simulink model "Problem16_BDsketch"  (R2020b)
settings: Solver=VariableStepAuto  StartTime=0.0  StopTime=10.0  RelTol=1e-3
values from neighbouring files (symbols this model uses):
  K_D = 2*zeta/omega_n * K_p - feff / kT    [problem12.m]    (also in problem13.m; problem15.m = (2*omega_n*zeta*tau_i + 1 - feff) ./ kT; problem16.m = (2*omega_n*zeta*tau_i + 1 - feff) ./ kT; problem17.m = (2*omega_n*zeta*tau_i + 1 - feff) ./ kT)
  K_I = omega_n^2 / kT    (= 1323.52941176)    [problem15.m]    (also in problem16.m = omega_n^2 / kT * ones(4,1); problem17.m = omega_n^2 / kT * ones(4,1); problem18.m; problem20.m = omega_n^2 / kT .* ones(4,1))
  kT = 0.17    [problem12.m]    (also in problem13.m; problem15.m; problem16.m; problem17.m)
  n = 53    [Problem7_9.m]    (also in Problem8_script.m = length(t); problem12.m; problem13.m; problem15.m)
undefined symbols (not defined in the file or in its folder): f_eff, J_eff, K_P
settings Model: Creator=Theis  LastModifiedBy=Theis

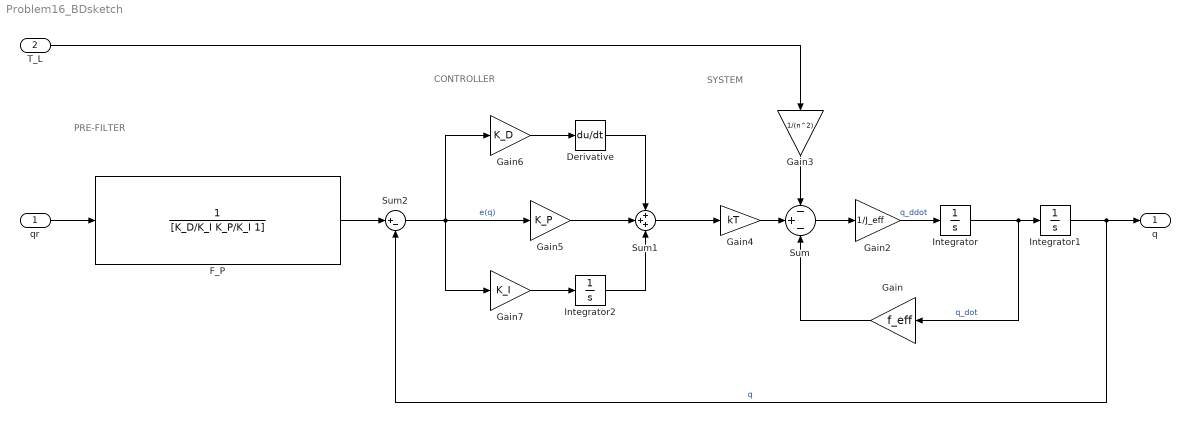
== system Problem16_BDsketch ==
  note: PRE-FILTER
  note: SYSTEM
  note: CONTROLLER
  qr : Inport
  T_L : Inport  Port=2
  Derivative : Derivative
  F_P : TransferFcn  Denominator=[K_D/K_I K_P/K_I 1]
  Gain : Gain  Gain=f_eff
  Gain2 : Gain  Gain=1/J_eff
  Gain3 : Gain  Gain=1/(n^2)
  Gain4 : Gain  Gain=kT
  Gain5 : Gain  Gain=K_P
  Gain6 : Gain  Gain=K_D
  Gain7 : Gain  Gain=K_I
  Integrator : Integrator
  Integrator1 : Integrator
  Integrator2 : Integrator
  Sum : Sum  Inputs=-+-
  Sum1 : Sum  Inputs=+++
  Sum2 : Sum  Inputs=|+-
  q : Outport
  wires:
  Integrator/1 -> Gain/1, Integrator1/1  "q_dot"
  Gain/1 -> Sum/3
  Gain2/1 -> Integrator/1  "q_ddot"
  Sum/1 -> Gain2/1
  T_L/1 -> Gain3/1
  Sum1/1 -> Gain4/1
  qr/1 -> F_P/1
  F_P/1 -> Sum2/1
  Integrator1/1 -> q/1, Sum2/2  "q"
  Gain5/1 -> Sum1/2
  Sum2/1 -> Gain6/1, Gain7/1, Gain5/1  "e(q)"
  Gain7/1 -> Integrator2/1
  Integrator2/1 -> Sum1/3
  Gain6/1 -> Derivative/1
  Derivative/1 -> Sum1/1
  Gain3/1 -> Sum/1
  Gain4/1 -> Sum/2
